simulink model "gm_case2mod_new"  (R2018b)
settings: Solver=FixedStepDiscrete  StartTime=0.0  StopTime=100000  FixedStep=1  RelTol=1e-3
(part 1 of 2)
settings Model: Creator=iris  LastModifiedBy=gvillanova
settings DataIOCC: LimitDataPoints=on  SaveFormat=Array  SignalLoggingSaveFormat=ModelDataLogs  SaveOutput=off  SignalLogging=off  SaveTime=off
settings OptimizationCC: BlockReduction=off  ConditionallyExecuteInputs=off  DefaultParameterBehavior=Inlined  ExpressionDepthLimit=2147483647  LifeSpan=inf
settings DebuggingCC: AlgebraicLoopMsg=error  UnderspecifiedInitializationDetection=Classic  MergeDetectMultiDrivingBlocksExec=none  SolverPrmCheckMsg=warning  InheritedTsInSrcMsg=none  SingleTaskRateTransMsg=error  FcnCallInpInsideContextMsg=warning  StateNameClashWarn=warning  SFUnexpectedBacktrackingDiag=warning  SFNoUnconditionalDefaultTransitionDiag=warning  SFExecutionAtInitializationDiag=none
settings HardwareCC: ProdBitPerPointer=32  ProdBitPerSizeT=32  ProdBitPerPtrDiffT=32  ProdLargestAtomicFloat=None  ProdIntDivRoundTo=Undefined  ProdEndianess=Unspecified  ProdWordSize=32  ProdHWDeviceType=ASIC/FPGA->ASIC/FPGA  ProdEqTarget=off
settings ModelReferenceCC: PropagateSignalLabelsOutOfModel=off
settings SFSimCC: SimUseLocalCustomCode=off
settings RTWCC: RTWUseLocalCustomCode=off
settings CodeAppCC: StateflowObjectComments=on
settings GRTTargetCC: TargetLangStandard=C89/C90 (ANSI)  GeneratePreprocessorConditionals=Disable all  CombineOutputUpdateFcns=off  GRTInterface=on
settings ConfigComp: CovMetricSettings=dw  CovHtmlReporting=on  CovSaveCumulativeToWorkspaceVar=on  CovSaveSingleToWorkspaceVar=on  CovExternalEMLEnable=off

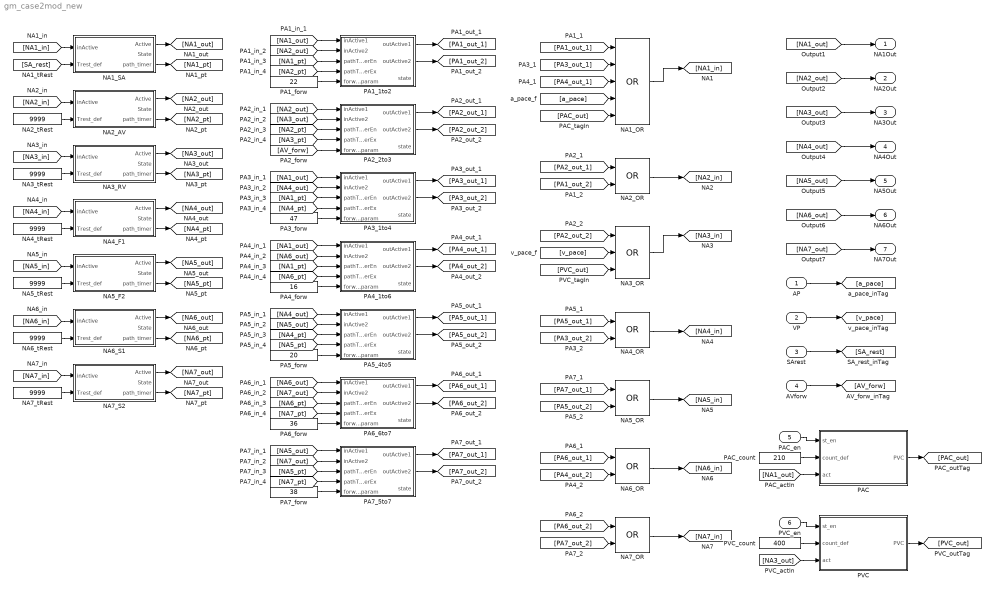
== system gm_case2mod_new ==
  AP : Inport  OutDataTypeStr=boolean  PortDimensions=1  SampleTime=1
  VP : Inport  Port=2  OutDataTypeStr=boolean  PortDimensions=1  SampleTime=1
  SArest : Inport  Port=3  OutDataTypeStr=uint16  PortDimensions=1  SampleTime=1
  AVforw : Inport  Port=4  OutDataTypeStr=uint16  PortDimensions=1  SampleTime=1
  PAC_en : Inport  Port=5  OutDataTypeStr=boolean  PortDimensions=1  SampleTime=1
  PVC_en : Inport  Port=6  OutDataTypeStr=boolean  PortDimensions=1  SampleTime=1
  NA1_OR : Logic  Operator=OR  Inputs=5  AllPortsSameDT=off  OutDataTypeStr=boolean
  NA1_SA : Subsystem  mask{TERP_s_m=double(200), TERP_defs_m=double(200), TRRP_s_m=double(100), TRRP_def_m=double(100), Trest_s_m=double(300), Terp_min_m=double(200), Terp_max_m=double(200)}
      mask prompts: TERP_s_m "Terp Start"; TERP_defs_m "Terp Default Start"; TRRP_s_m "Trrp Start"; TRRP_def_m "Trrp Default"; Trest_s_m "Trest Start"; Terp_min_m "Terp Min"; Terp_max_m "Terp Max"
  NA2_AV : Subsystem  mask{TERP_s_m=double(200), TERP_defs_m=double(200), TRRP_s_m=double(100), TRRP_def_m=double(100), Trest_s_m=double(9999), Terp_min_m=double(200), Terp_max_m=double(200)}
      mask prompts: TERP_s_m "Terp Start"; TERP_defs_m "Terp Default Start"; TRRP_s_m "Trrp Start"; TRRP_def_m "Trrp Default"; Trest_s_m "Trest Start"; Terp_min_m "Terp Min"; Terp_max_m "Terp Max"
  NA2_OR : Logic  Operator=OR  AllPortsSameDT=off  OutDataTypeStr=boolean
  NA2_tRest : Constant  Value=9999  OutDataTypeStr=uint16
  NA3_OR : Logic  Operator=OR  Inputs=3  AllPortsSameDT=off  OutDataTypeStr=boolean
  NA3_RV : Subsystem  mask{TERP_s_m=double(250), TERP_defs_m=double(250), TRRP_s_m=double(100), TRRP_def_m=double(100), Trest_s_m=double(9999), Terp_min_m=double(250), Terp_max_m=double(250)}
      mask prompts: TERP_s_m "Terp Start"; TERP_defs_m "Terp Default Start"; TRRP_s_m "Trrp Start"; TRRP_def_m "Trrp Default"; Trest_s_m "Trest Start"; Terp_min_m "Terp Min"; Terp_max_m "Terp Max"
  NA3_tRest : Constant  Value=9999  OutDataTypeStr=uint16
  NA4_F1 : Subsystem  mask{TERP_s_m=double(250), TERP_defs_m=double(250), TRRP_s_m=double(100), TRRP_def_m=double(100), Trest_s_m=double(9999), Terp_min_m=double(250), Terp_max_m=double(250)}
      mask prompts: TERP_s_m "Terp Start"; TERP_defs_m "Terp Default Start"; TRRP_s_m "Trrp Start"; TRRP_def_m "Trrp Default"; Trest_s_m "Trest Start"; Terp_min_m "Terp Min"; Terp_max_m "Terp Max"
  NA4_OR : Logic  Operator=OR  AllPortsSameDT=off  OutDataTypeStr=boolean
  NA4_tRest : Constant  Value=9999  OutDataTypeStr=uint16
  NA5_F2 : Subsystem  mask{TERP_s_m=double(250), TERP_defs_m=double(250), TRRP_s_m=double(100), TRRP_def_m=double(100), Trest_s_m=double(9999), Terp_min_m=double(250), Terp_max_m=double(250)}
      mask prompts: TERP_s_m "Terp Start"; TERP_defs_m "Terp Default Start"; TRRP_s_m "Trrp Start"; TRRP_def_m "Trrp Default"; Trest_s_m "Trest Start"; Terp_min_m "Terp Min"; Terp_max_m "Terp Max"
  NA5_OR : Logic  Operator=OR  AllPortsSameDT=off  OutDataTypeStr=boolean
  NA5_tRest : Constant  Value=9999  OutDataTypeStr=uint16
  NA6_OR : Logic  Operator=OR  AllPortsSameDT=off  OutDataTypeStr=boolean
  NA6_S1 : Subsystem  mask{TERP_s_m=double(150), TERP_defs_m=double(150), TRRP_s_m=double(100), TRRP_def_m=double(100), Trest_s_m=double(9999), Terp_min_m=double(150), Terp_max_m=double(150)}
      mask prompts: TERP_s_m "Terp Start"; TERP_defs_m "Terp Default Start"; TRRP_s_m "Trrp Start"; TRRP_def_m "Trrp Default"; Trest_s_m "Trest Start"; Terp_min_m "Terp Min"; Terp_max_m "Terp Max"
  NA6_tRest : Constant  Value=9999  OutDataTypeStr=uint16
  NA7_OR : Logic  Operator=OR  AllPortsSameDT=off  OutDataTypeStr=boolean
  NA7_S2 : Subsystem  mask{TERP_s_m=double(150), TERP_defs_m=double(150), TRRP_s_m=double(100), TRRP_def_m=double(100), Trest_s_m=double(9999), Terp_min_m=double(150), Terp_max_m=double(150)}
      mask prompts: TERP_s_m "Terp Start"; TERP_defs_m "Terp Default Start"; TRRP_s_m "Trrp Start"; TRRP_def_m "Trrp Default"; Trest_s_m "Trest Start"; Terp_min_m "Terp Min"; Terp_max_m "Terp Max"
  NA7_tRest : Constant  Value=9999  OutDataTypeStr=uint16
  PA1_1to2 : Subsystem  mask{min_path_par_m=double(10), bck_param_m=double(132)}
      mask prompts: min_path_par_m "Min Path Param"; bck_param_m "Back Param"
  PA1_forw : Constant  Value=22  OutDataTypeStr=uint16
  PA2_2to3 : Subsystem  mask{min_path_par_m=double(90), bck_param_m=double(144)}
      mask prompts: min_path_par_m "Min Path Param"; bck_param_m "Back Param"
  PA3_1to4 : Subsystem  mask{min_path_par_m=double(10), bck_param_m=double(32767)}
      mask prompts: min_path_par_m "Min Path Param"; bck_param_m "Back Param"
  PA3_forw : Constant  Value=47  OutDataTypeStr=uint16
  PA4_1to6 : Subsystem  mask{min_path_par_m=double(80), bck_param_m=double(16)}
      mask prompts: min_path_par_m "Min Path Param"; bck_param_m "Back Param"
  PA4_forw : Constant  Value=16  OutDataTypeStr=uint16
  PA5_4to5 : Subsystem  mask{min_path_par_m=double(50), bck_param_m=double(20)}
      mask prompts: min_path_par_m "Min Path Param"; bck_param_m "Back Param"
  PA5_forw : Constant  Value=20  OutDataTypeStr=uint16
  PA6_6to7 : Subsystem  mask{min_path_par_m=double(100), bck_param_m=double(36)}
      mask prompts: min_path_par_m "Min Path Param"; bck_param_m "Back Param"
  PA6_forw : Constant  Value=36  OutDataTypeStr=uint16
  PA7_5to7 : Subsystem  mask{min_path_par_m=double(50), bck_param_m=double(38)}
      mask prompts: min_path_par_m "Min Path Param"; bck_param_m "Back Param"
  PA7_forw : Constant  Value=38  OutDataTypeStr=uint16
  PAC : Subsystem
  PAC_count : Constant  Value=210  OutDataTypeStr=uint16
  PVC : Subsystem
  PVC_count : Constant  Value=400  OutDataTypeStr=uint16
  NA1Out : Outport
  NA2Out : Outport  Port=2
  NA3Out : Outport  Port=3
  NA4Out : Outport  Port=4
  NA5Out : Outport  Port=5
  NA6Out : Outport  Port=6
  NA7Out : Outport  Port=7
  wires:
  AP/1 -> [a_pace]
  VP/1 -> [v_pace]
  SArest/1 -> [SA_rest]
  AVforw/1 -> [AV_forw]
  PAC_en/1 -> PAC/1(st_en)
  PVC_en/1 -> PVC/1(st_en)
  NA1_OR/1 -> [NA1_in]
  NA1_SA/1(Active) -> [NA1_out]
  NA1_SA/3(path_timer) -> [NA1_pt]
  [NA1_in] -> NA1_SA/1(inActive)
  [SA_rest] -> NA1_SA/2(Trest_def)
  NA2_AV/1(Active) -> [NA2_out]
  NA2_AV/3(path_timer) -> [NA2_pt]
  NA2_OR/1 -> [NA2_in]
  [NA2_in] -> NA2_AV/1(inActive)
  NA2_tRest/1 -> NA2_AV/2(Trest_def)
  NA3_OR/1 -> [NA3_in]
  NA3_RV/1(Active) -> [NA3_out]
  NA3_RV/3(path_timer) -> [NA3_pt]
  [NA3_in] -> NA3_RV/1(inActive)
  NA3_tRest/1 -> NA3_RV/2(Trest_def)
  NA4_F1/1(Active) -> [NA4_out]
  NA4_F1/3(path_timer) -> [NA4_pt]
  NA4_OR/1 -> [NA4_in]
  [NA4_in] -> NA4_F1/1(inActive)
  NA4_tRest/1 -> NA4_F1/2(Trest_def)
  NA5_F2/1(Active) -> [NA5_out]
  NA5_F2/3(path_timer) -> [NA5_pt]
  NA5_OR/1 -> [NA5_in]
  [NA5_in] -> NA5_F2/1(inActive)
  NA5_tRest/1 -> NA5_F2/2(Trest_def)
  NA6_OR/1 -> [NA6_in]
  NA6_S1/1(Active) -> [NA6_out]
  NA6_S1/3(path_timer) -> [NA6_pt]
  [NA6_in] -> NA6_S1/1(inActive)
  NA6_tRest/1 -> NA6_S1/2(Trest_def)
  NA7_OR/1 -> [NA7_in]
  NA7_S2/1(Active) -> [NA7_out]
  NA7_S2/3(path_timer) -> [NA7_pt]
  [NA7_in] -> NA7_S2/1(inActive)
  NA7_tRest/1 -> NA7_S2/2(Trest_def)
  [NA1_out] -> NA1Out/1
  [NA2_out] -> NA2Out/1
  [NA3_out] -> NA3Out/1
  [NA4_out] -> NA4Out/1
  [NA5_out] -> NA5Out/1
  [NA6_out] -> NA6Out/1
  [NA7_out] -> NA7Out/1
  [PA1_out_1] -> NA1_OR/1
  PA1_1to2/1(outActive1) -> [PA1_out_1]
  PA1_1to2/2(outActive2) -> [PA1_out_2]
  [PA1_out_2] -> NA2_OR/2
  PA1_forw/1 -> PA1_1to2/5(forw_param)
  [NA1_out] -> PA1_1to2/1(inActive1)
  [NA2_out] -> PA1_1to2/2(inActive2)
  [NA1_pt] -> PA1_1to2/3(pathTimerEn)
  [NA2_pt] -> PA1_1to2/4(pathTimerEx)
  [PA2_out_1] -> NA2_OR/1
  [PA2_out_2] -> NA3_OR/1
  PA2_2to3/1(outActive1) -> [PA2_out_1]
  PA2_2to3/2(outActive2) -> [PA2_out_2]
  [AV_forw] -> PA2_2to3/5(forw_param)
  [NA2_out] -> PA2_2to3/1(inActive1)
  [NA3_out] -> PA2_2to3/2(inActive2)
  [NA2_pt] -> PA2_2to3/3(pathTimerEn)
  [NA3_pt] -> PA2_2to3/4(pathTimerEx)
  [PA3_out_1] -> NA1_OR/2
  PA3_1to4/1(outActive1) -> [PA3_out_1]
  PA3_1to4/2(outActive2) -> [PA3_out_2]
  [PA3_out_2] -> NA4_OR/2
  PA3_forw/1 -> PA3_1to4/5(forw_param)
  [NA1_out] -> PA3_1to4/1(inActive1)
  [NA4_out] -> PA3_1to4/2(inActive2)
  [NA1_pt] -> PA3_1to4/3(pathTimerEn)
  [NA4_pt] -> PA3_1to4/4(pathTimerEx)
  [PA4_out_1] -> NA1_OR/3
  PA4_1to6/1(outActive1) -> [PA4_out_1]
  PA4_1to6/2(outActive2) -> [PA4_out_2]
  [PA4_out_2] -> NA6_OR/2
  PA4_forw/1 -> PA4_1to6/5(forw_param)
  [NA1_out] -> PA4_1to6/1(inActive1)
  [NA6_out] -> PA4_1to6/2(inActive2)
  [NA1_pt] -> PA4_1to6/3(pathTimerEn)
  [NA6_pt] -> PA4_1to6/4(pathTimerEx)
  [PA5_out_1] -> NA4_OR/1
  [PA5_out_2] -> NA5_OR/2
  PA5_4to5/1(outActive1) -> [PA5_out_1]
  PA5_4to5/2(outActive2) -> [PA5_out_2]
  PA5_forw/1 -> PA5_4to5/5(forw_param)
  [NA4_out] -> PA5_4to5/1(inActive1)
  [NA5_out] -> PA5_4to5/2(inActive2)
  [NA4_pt] -> PA5_4to5/3(pathTimerEn)
  [NA5_pt] -> PA5_4to5/4(pathTimerEx)
  [PA6_out_1] -> NA6_OR/1
  [PA6_out_2] -> NA7_OR/1
  PA6_6to7/1(outActive1) -> [PA6_out_1]
  PA6_6to7/2(outActive2) -> [PA6_out_2]
  PA6_forw/1 -> PA6_6to7/5(forw_param)
  [NA6_out] -> PA6_6to7/1(inActive1)
  [NA7_out] -> PA6_6to7/2(inActive2)
  [NA6_pt] -> PA6_6to7/3(pathTimerEn)
  [NA7_pt] -> PA6_6to7/4(pathTimerEx)
  [PA7_out_1] -> NA5_OR/1
  [PA7_out_2] -> NA7_OR/2
  PA7_5to7/1(outActive1) -> [PA7_out_1]
  PA7_5to7/2(outActive2) -> [PA7_out_2]
  PA7_forw/1 -> PA7_5to7/5(forw_param)
  [NA5_out] -> PA7_5to7/1(inActive1)
  [NA7_out] -> PA7_5to7/2(inActive2)
  [NA5_pt] -> PA7_5to7/3(pathTimerEn)
  [NA7_pt] -> PA7_5to7/4(pathTimerEx)
  PAC/1(PVC) -> [PAC_out]
  [NA1_out] -> PAC/3(act)
  PAC_count/1 -> PAC/2(count_def)
  [PAC_out] -> NA1_OR/5
  PVC/1(PVC) -> [PVC_out]
  [NA3_out] -> PVC/3(act)
  PVC_count/1 -> PVC/2(count_def)
  [PVC_out] -> NA3_OR/3
  [a_pace] -> NA1_OR/4
  [v_pace] -> NA3_OR/2

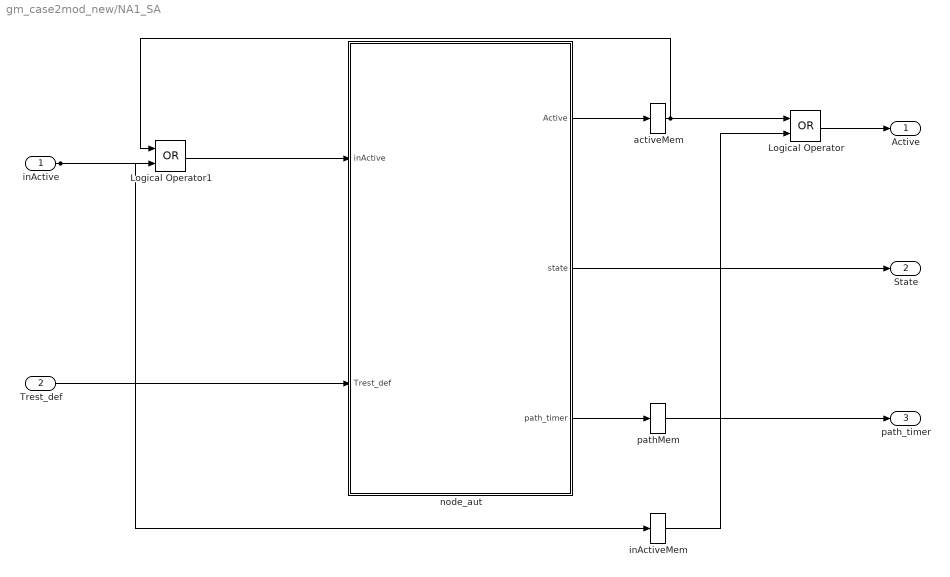
== system gm_case2mod_new/NA1_SA ==
  inActive : Inport  OutDataTypeStr=boolean  SampleTime=1
  Trest_def : Inport  Port=2  OutDataTypeStr=uint16  SampleTime=1
  Logical Operator : Logic  Operator=OR  AllPortsSameDT=off  OutDataTypeStr=boolean
  Logical Operator1 : Logic  Operator=OR  AllPortsSameDT=off  OutDataTypeStr=boolean
  activeMem : Memory  InheritSampleTime=on
  inActiveMem : Memory  InheritSampleTime=on
  node_aut : Subsystem
  pathMem : Memory  InheritSampleTime=on
  Active : Outport
  State : Outport  Port=2
  path_timer : Outport  Port=3
  wires:
  inActive/1 -> Logical Operator1/2, inActiveMem/1
  Trest_def/1 -> node_aut/2(Trest_def)
  Logical Operator/1 -> Active/1
  Logical Operator1/1 -> node_aut/1(inActive)
  activeMem/1 -> Logical Operator1/1, Logical Operator/1
  inActiveMem/1 -> Logical Operator/2
  node_aut/1(Active) -> activeMem/1
  node_aut/2(state) -> State/1
  node_aut/3(path_timer) -> pathMem/1
  pathMem/1 -> path_timer/1

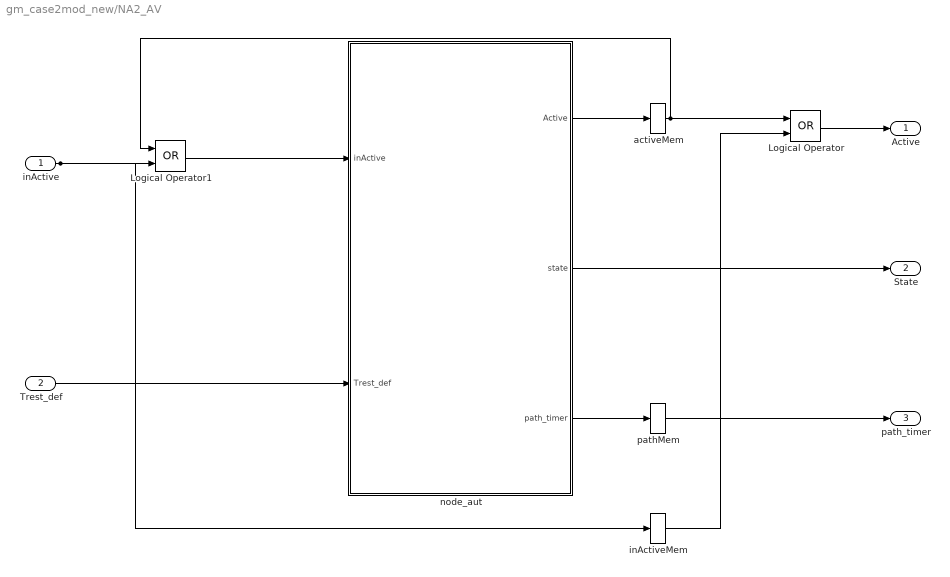
== system gm_case2mod_new/NA2_AV ==
  inActive : Inport  OutDataTypeStr=boolean  SampleTime=1
  Trest_def : Inport  Port=2  OutDataTypeStr=uint16
  Logical Operator : Logic  Operator=OR  AllPortsSameDT=off  OutDataTypeStr=boolean
  Logical Operator1 : Logic  Operator=OR  AllPortsSameDT=off  OutDataTypeStr=boolean
  activeMem : Memory  InheritSampleTime=on
  inActiveMem : Memory  InheritSampleTime=on
  node_aut : Subsystem
  pathMem : Memory  InheritSampleTime=on
  Active : Outport
  State : Outport  Port=2
  path_timer : Outport  Port=3
  wires:
  inActive/1 -> Logical Operator1/2, inActiveMem/1
  Trest_def/1 -> node_aut/2(Trest_def)
  Logical Operator/1 -> Active/1
  Logical Operator1/1 -> node_aut/1(inActive)
  activeMem/1 -> Logical Operator1/1, Logical Operator/1
  inActiveMem/1 -> Logical Operator/2
  node_aut/1(Active) -> activeMem/1
  node_aut/2(state) -> State/1
  node_aut/3(path_timer) -> pathMem/1
  pathMem/1 -> path_timer/1

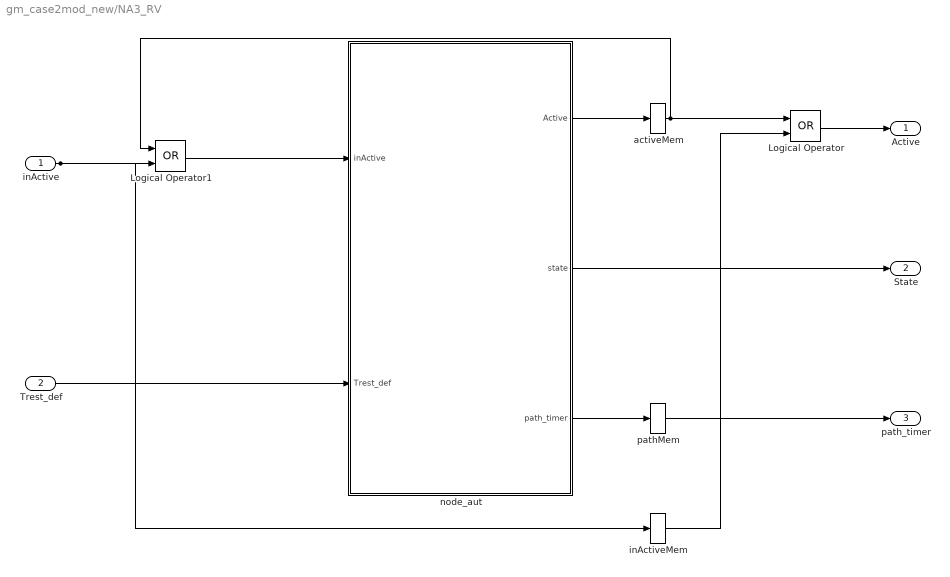
== system gm_case2mod_new/NA3_RV ==
  inActive : Inport  OutDataTypeStr=boolean  SampleTime=1
  Trest_def : Inport  Port=2  OutDataTypeStr=uint16
  Logical Operator : Logic  Operator=OR  AllPortsSameDT=off  OutDataTypeStr=boolean
  Logical Operator1 : Logic  Operator=OR  AllPortsSameDT=off  OutDataTypeStr=boolean
  activeMem : Memory  InheritSampleTime=on
  inActiveMem : Memory  InheritSampleTime=on
  node_aut : Subsystem
  pathMem : Memory  InheritSampleTime=on
  Active : Outport
  State : Outport  Port=2
  path_timer : Outport  Port=3
  wires:
  inActive/1 -> Logical Operator1/2, inActiveMem/1
  Trest_def/1 -> node_aut/2(Trest_def)
  Logical Operator/1 -> Active/1
  Logical Operator1/1 -> node_aut/1(inActive)
  activeMem/1 -> Logical Operator1/1, Logical Operator/1
  inActiveMem/1 -> Logical Operator/2
  node_aut/1(Active) -> activeMem/1
  node_aut/2(state) -> State/1
  node_aut/3(path_timer) -> pathMem/1
  pathMem/1 -> path_timer/1

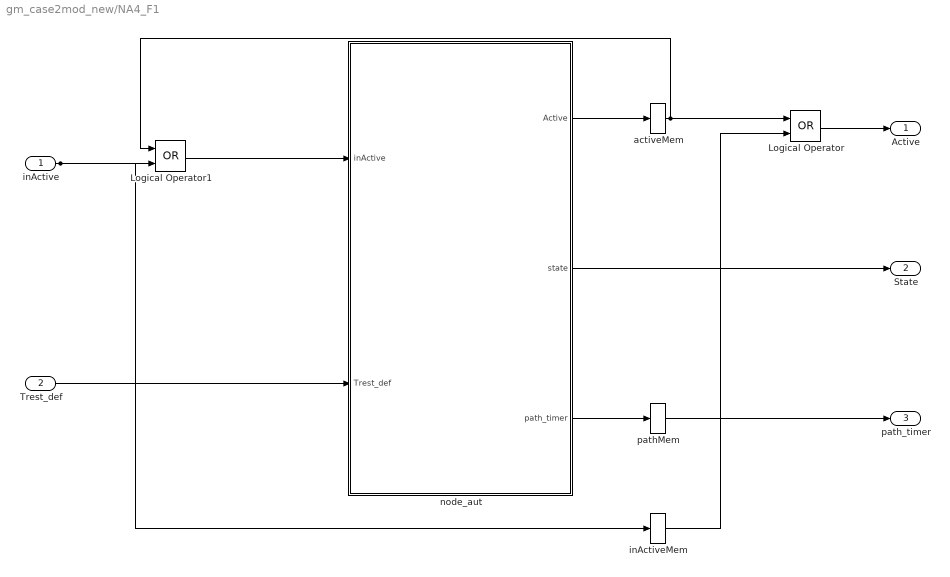
== system gm_case2mod_new/NA4_F1 ==
  inActive : Inport  OutDataTypeStr=boolean  SampleTime=1
  Trest_def : Inport  Port=2  OutDataTypeStr=uint16
  Logical Operator : Logic  Operator=OR  AllPortsSameDT=off  OutDataTypeStr=boolean
  Logical Operator1 : Logic  Operator=OR  AllPortsSameDT=off  OutDataTypeStr=boolean
  activeMem : Memory  InheritSampleTime=on
  inActiveMem : Memory  InheritSampleTime=on
  node_aut : Subsystem
  pathMem : Memory  InheritSampleTime=on
  Active : Outport
  State : Outport  Port=2
  path_timer : Outport  Port=3
  wires:
  inActive/1 -> Logical Operator1/2, inActiveMem/1
  Trest_def/1 -> node_aut/2(Trest_def)
  Logical Operator/1 -> Active/1
  Logical Operator1/1 -> node_aut/1(inActive)
  activeMem/1 -> Logical Operator1/1, Logical Operator/1
  inActiveMem/1 -> Logical Operator/2
  node_aut/1(Active) -> activeMem/1
  node_aut/2(state) -> State/1
  node_aut/3(path_timer) -> pathMem/1
  pathMem/1 -> path_timer/1

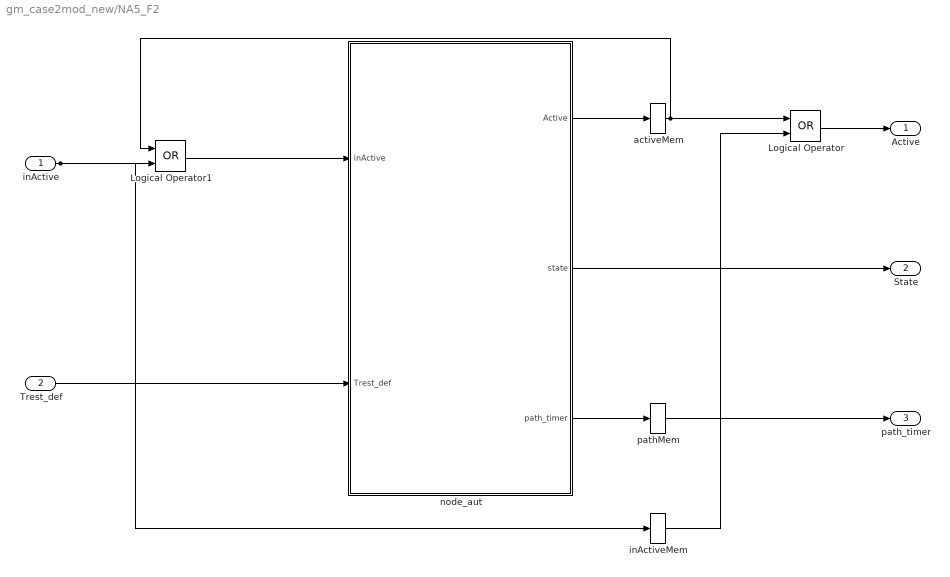
== system gm_case2mod_new/NA5_F2 ==
  inActive : Inport  OutDataTypeStr=boolean  SampleTime=1
  Trest_def : Inport  Port=2  OutDataTypeStr=uint16
  Logical Operator : Logic  Operator=OR  AllPortsSameDT=off  OutDataTypeStr=boolean
  Logical Operator1 : Logic  Operator=OR  AllPortsSameDT=off  OutDataTypeStr=boolean
  activeMem : Memory  InheritSampleTime=on
  inActiveMem : Memory  InheritSampleTime=on
  node_aut : Subsystem
  pathMem : Memory  InheritSampleTime=on
  Active : Outport
  State : Outport  Port=2
  path_timer : Outport  Port=3
  wires:
  inActive/1 -> Logical Operator1/2, inActiveMem/1
  Trest_def/1 -> node_aut/2(Trest_def)
  Logical Operator/1 -> Active/1
  Logical Operator1/1 -> node_aut/1(inActive)
  activeMem/1 -> Logical Operator1/1, Logical Operator/1
  inActiveMem/1 -> Logical Operator/2
  node_aut/1(Active) -> activeMem/1
  node_aut/2(state) -> State/1
  node_aut/3(path_timer) -> pathMem/1
  pathMem/1 -> path_timer/1

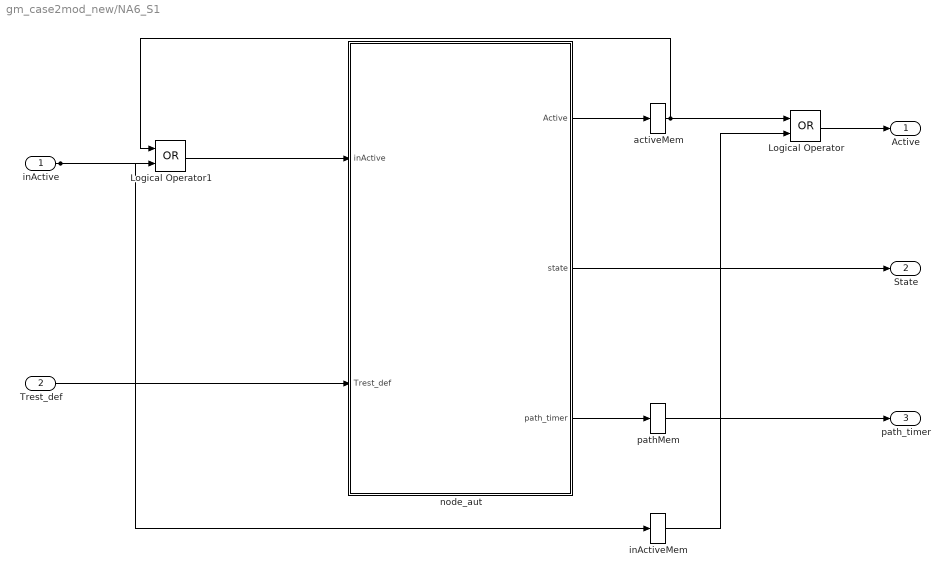
== system gm_case2mod_new/NA6_S1 ==
  inActive : Inport  OutDataTypeStr=boolean  SampleTime=1
  Trest_def : Inport  Port=2  OutDataTypeStr=uint16
  Logical Operator : Logic  Operator=OR  AllPortsSameDT=off  OutDataTypeStr=boolean
  Logical Operator1 : Logic  Operator=OR  AllPortsSameDT=off  OutDataTypeStr=boolean
  activeMem : Memory  InheritSampleTime=on
  inActiveMem : Memory  InheritSampleTime=on
  node_aut : Subsystem
  pathMem : Memory  InheritSampleTime=on
  Active : Outport
  State : Outport  Port=2
  path_timer : Outport  Port=3
  wires:
  inActive/1 -> Logical Operator1/2, inActiveMem/1
  Trest_def/1 -> node_aut/2(Trest_def)
  Logical Operator/1 -> Active/1
  Logical Operator1/1 -> node_aut/1(inActive)
  activeMem/1 -> Logical Operator1/1, Logical Operator/1
  inActiveMem/1 -> Logical Operator/2
  node_aut/1(Active) -> activeMem/1
  node_aut/2(state) -> State/1
  node_aut/3(path_timer) -> pathMem/1
  pathMem/1 -> path_timer/1

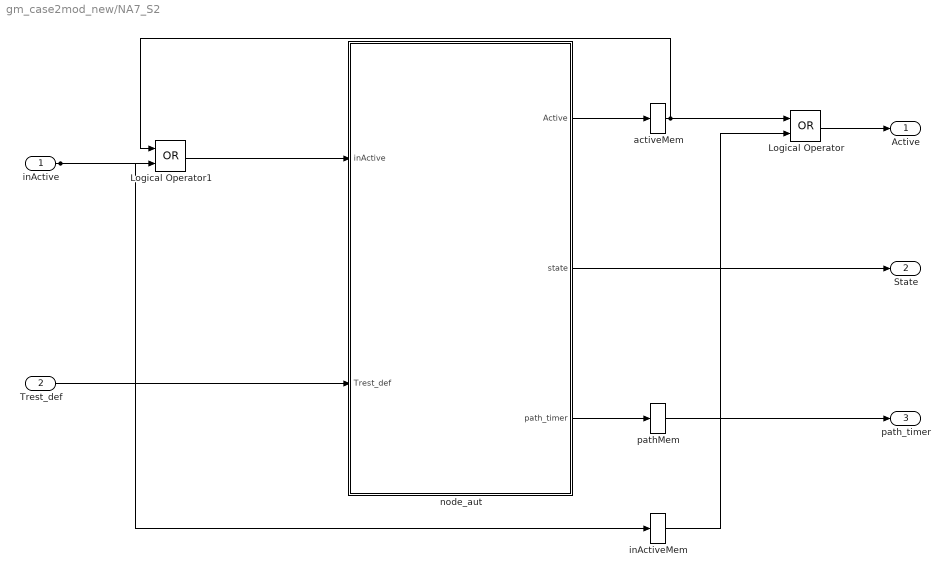
== system gm_case2mod_new/NA7_S2 ==
  inActive : Inport  OutDataTypeStr=boolean  SampleTime=1
  Trest_def : Inport  Port=2  OutDataTypeStr=uint16
  Logical Operator : Logic  Operator=OR  AllPortsSameDT=off  OutDataTypeStr=boolean
  Logical Operator1 : Logic  Operator=OR  AllPortsSameDT=off  OutDataTypeStr=boolean
  activeMem : Memory  InheritSampleTime=on
  inActiveMem : Memory  InheritSampleTime=on
  node_aut : Subsystem
  pathMem : Memory  InheritSampleTime=on
  Active : Outport
  State : Outport  Port=2
  path_timer : Outport  Port=3
  wires:
  inActive/1 -> Logical Operator1/2, inActiveMem/1
  Trest_def/1 -> node_aut/2(Trest_def)
  Logical Operator/1 -> Active/1
  Logical Operator1/1 -> node_aut/1(inActive)
  activeMem/1 -> Logical Operator1/1, Logical Operator/1
  inActiveMem/1 -> Logical Operator/2
  node_aut/1(Active) -> activeMem/1
  node_aut/2(state) -> State/1
  node_aut/3(path_timer) -> pathMem/1
  pathMem/1 -> path_timer/1

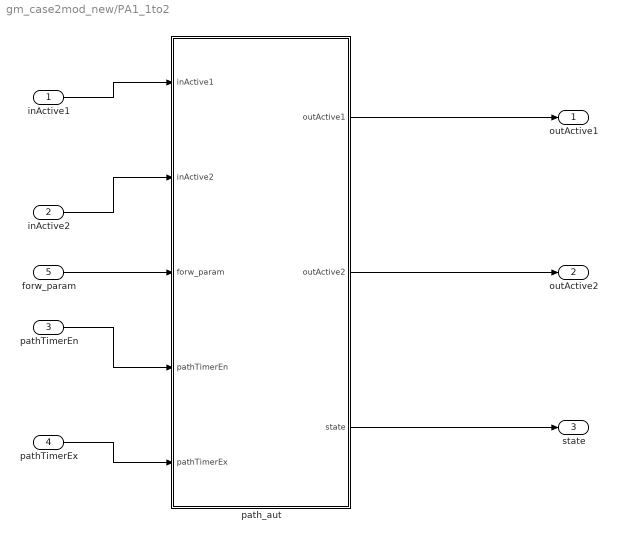
== system gm_case2mod_new/PA1_1to2 ==
  inActive1 : Inport  OutDataTypeStr=boolean  SampleTime=1
  inActive2 : Inport  Port=2  OutDataTypeStr=boolean  SampleTime=1
  pathTimerEn : Inport  Port=3  OutDataTypeStr=uint16  SampleTime=1
  pathTimerEx : Inport  Port=4  OutDataTypeStr=uint16  SampleTime=1
  forw_param : Inport  Port=5  OutDataTypeStr=uint16
  path_aut : Subsystem
  outActive1 : Outport
  outActive2 : Outport  Port=2
  state : Outport  Port=3
  wires:
  inActive1/1 -> path_aut/1(inActive1)
  inActive2/1 -> path_aut/2(inActive2)
  pathTimerEn/1 -> path_aut/4(pathTimerEn)
  pathTimerEx/1 -> path_aut/5(pathTimerEx)
  forw_param/1 -> path_aut/3(forw_param)
  path_aut/1(outActive1) -> outActive1/1
  path_aut/2(outActive2) -> outActive2/1
  path_aut/3(state) -> state/1

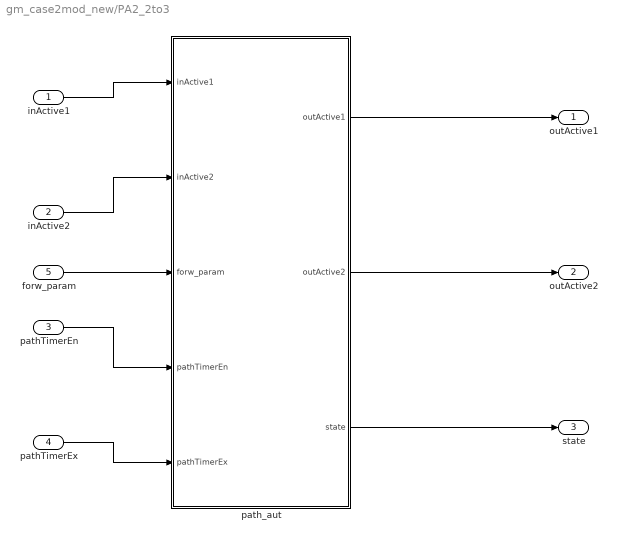
== system gm_case2mod_new/PA2_2to3 ==
  inActive1 : Inport  OutDataTypeStr=boolean  SampleTime=1
  inActive2 : Inport  Port=2  OutDataTypeStr=boolean  SampleTime=1
  pathTimerEn : Inport  Port=3  OutDataTypeStr=uint16  SampleTime=1
  pathTimerEx : Inport  Port=4  OutDataTypeStr=uint16  SampleTime=1
  forw_param : Inport  Port=5  OutDataTypeStr=uint16  SampleTime=1
  path_aut : Subsystem
  outActive1 : Outport
  outActive2 : Outport  Port=2
  state : Outport  Port=3
  wires:
  inActive1/1 -> path_aut/1(inActive1)
  inActive2/1 -> path_aut/2(inActive2)
  pathTimerEn/1 -> path_aut/4(pathTimerEn)
  pathTimerEx/1 -> path_aut/5(pathTimerEx)
  forw_param/1 -> path_aut/3(forw_param)
  path_aut/1(outActive1) -> outActive1/1
  path_aut/2(outActive2) -> outActive2/1
  path_aut/3(state) -> state/1

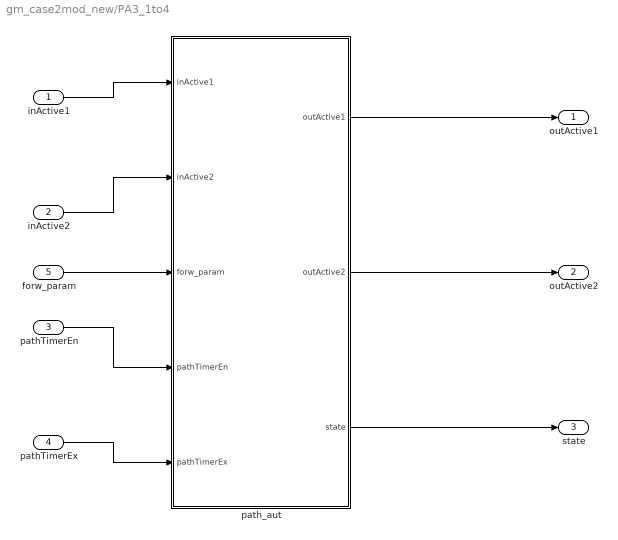
== system gm_case2mod_new/PA3_1to4 ==
  inActive1 : Inport  OutDataTypeStr=boolean  SampleTime=1
  inActive2 : Inport  Port=2  OutDataTypeStr=boolean  SampleTime=1
  pathTimerEn : Inport  Port=3  OutDataTypeStr=uint16  SampleTime=1
  pathTimerEx : Inport  Port=4  OutDataTypeStr=uint16  SampleTime=1
  forw_param : Inport  Port=5  OutDataTypeStr=uint16
  path_aut : Subsystem
  outActive1 : Outport
  outActive2 : Outport  Port=2
  state : Outport  Port=3
  wires:
  inActive1/1 -> path_aut/1(inActive1)
  inActive2/1 -> path_aut/2(inActive2)
  pathTimerEn/1 -> path_aut/4(pathTimerEn)
  pathTimerEx/1 -> path_aut/5(pathTimerEx)
  forw_param/1 -> path_aut/3(forw_param)
  path_aut/1(outActive1) -> outActive1/1
  path_aut/2(outActive2) -> outActive2/1
  path_aut/3(state) -> state/1

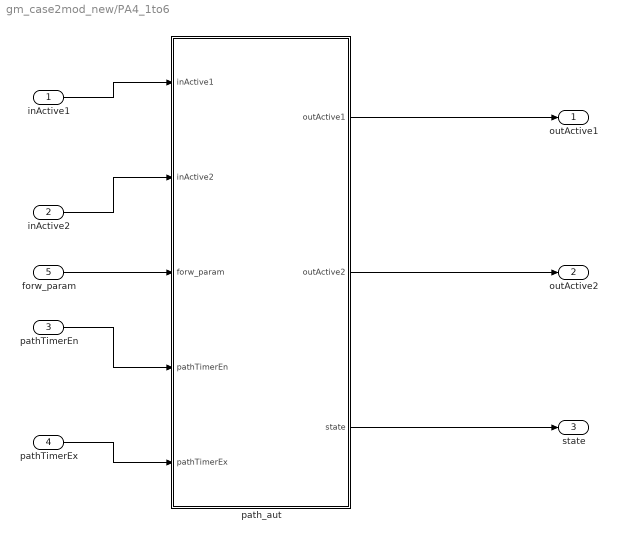
== system gm_case2mod_new/PA4_1to6 ==
  inActive1 : Inport  OutDataTypeStr=boolean  SampleTime=1
  inActive2 : Inport  Port=2  OutDataTypeStr=boolean  SampleTime=1
  pathTimerEn : Inport  Port=3  OutDataTypeStr=uint16  SampleTime=1
  pathTimerEx : Inport  Port=4  OutDataTypeStr=uint16  SampleTime=1
  forw_param : Inport  Port=5  OutDataTypeStr=uint16
  path_aut : Subsystem
  outActive1 : Outport
  outActive2 : Outport  Port=2
  state : Outport  Port=3
  wires:
  inActive1/1 -> path_aut/1(inActive1)
  inActive2/1 -> path_aut/2(inActive2)
  pathTimerEn/1 -> path_aut/4(pathTimerEn)
  pathTimerEx/1 -> path_aut/5(pathTimerEx)
  forw_param/1 -> path_aut/3(forw_param)
  path_aut/1(outActive1) -> outActive1/1
  path_aut/2(outActive2) -> outActive2/1
  path_aut/3(state) -> state/1

== system gm_case2mod_new/PA5_4to5 ==
  inActive1 : Inport  OutDataTypeStr=boolean  SampleTime=1
  inActive2 : Inport  Port=2  OutDataTypeStr=boolean  SampleTime=1
  pathTimerEn : Inport  Port=3  OutDataTypeStr=uint16  SampleTime=1
  pathTimerEx : Inport  Port=4  OutDataTypeStr=uint16  SampleTime=1
  forw_param : Inport  Port=5  OutDataTypeStr=uint16
  path_aut : Subsystem
  outActive1 : Outport
  outActive2 : Outport  Port=2
  state : Outport  Port=3
  wires:
  inActive1/1 -> path_aut/1(inActive1)
  inActive2/1 -> path_aut/2(inActive2)
  pathTimerEn/1 -> path_aut/4(pathTimerEn)
  pathTimerEx/1 -> path_aut/5(pathTimerEx)
  forw_param/1 -> path_aut/3(forw_param)
  path_aut/1(outActive1) -> outActive1/1
  path_aut/2(outActive2) -> outActive2/1
  path_aut/3(state) -> state/1

== system gm_case2mod_new/PA6_6to7 ==
  inActive1 : Inport  OutDataTypeStr=boolean  SampleTime=1
  inActive2 : Inport  Port=2  OutDataTypeStr=boolean  SampleTime=1
  pathTimerEn : Inport  Port=3  OutDataTypeStr=uint16  SampleTime=1
  pathTimerEx : Inport  Port=4  OutDataTypeStr=uint16  SampleTime=1
  forw_param : Inport  Port=5  OutDataTypeStr=uint16
  path_aut : Subsystem
  outActive1 : Outport
  outActive2 : Outport  Port=2
  state : Outport  Port=3
  wires:
  inActive1/1 -> path_aut/1(inActive1)
  inActive2/1 -> path_aut/2(inActive2)
  pathTimerEn/1 -> path_aut/4(pathTimerEn)
  pathTimerEx/1 -> path_aut/5(pathTimerEx)
  forw_param/1 -> path_aut/3(forw_param)
  path_aut/1(outActive1) -> outActive1/1
  path_aut/2(outActive2) -> outActive2/1
  path_aut/3(state) -> state/1

== system gm_case2mod_new/PA7_5to7 ==
  inActive1 : Inport  OutDataTypeStr=boolean  SampleTime=1
  inActive2 : Inport  Port=2  OutDataTypeStr=boolean  SampleTime=1
  pathTimerEn : Inport  Port=3  OutDataTypeStr=uint16  SampleTime=1
  pathTimerEx : Inport  Port=4  OutDataTypeStr=uint16  SampleTime=1
  forw_param : Inport  Port=5  OutDataTypeStr=uint16
  path_aut : Subsystem
  outActive1 : Outport
  outActive2 : Outport  Port=2
  state : Outport  Port=3
  wires:
  inActive1/1 -> path_aut/1(inActive1)
  inActive2/1 -> path_aut/2(inActive2)
  pathTimerEn/1 -> path_aut/4(pathTimerEn)
  pathTimerEx/1 -> path_aut/5(pathTimerEx)
  forw_param/1 -> path_aut/3(forw_param)
  path_aut/1(outActive1) -> outActive1/1
  path_aut/2(outActive2) -> outActive2/1
  path_aut/3(state) -> state/1

== system gm_case2mod_new/PAC ==
  st_en : Inport  OutDataTypeStr=boolean  SampleTime=1
  count_def : Inport  Port=2  OutDataTypeStr=uint16
  act : Inport  Port=3  OutDataTypeStr=boolean  SampleTime=1
  SimpleModeling_c8_PVC : Stateflow chart  TreatAsAtomicUnit=on
  PVC : Outport
  wires:
  st_en/1 -> SimpleModeling_c8_PVC/1(st_en)
  count_def/1 -> SimpleModeling_c8_PVC/2(count_def)
  act/1 -> SimpleModeling_c8_PVC/3(act)
  SimpleModeling_c8_PVC/1(PVC) -> PVC/1

== system gm_case2mod_new/PVC ==
  st_en : Inport  OutDataTypeStr=boolean  SampleTime=1
  count_def : Inport  Port=2  OutDataTypeStr=uint16
  act : Inport  Port=3  OutDataTypeStr=boolean  SampleTime=1
  SimpleModeling_c8_PVC : Stateflow chart  TreatAsAtomicUnit=on
  PVC : Outport
  wires:
  SimpleModeling_c8_PVC/1(PVC) -> PVC/1
  act/1 -> SimpleModeling_c8_PVC/3(act)
  count_def/1 -> SimpleModeling_c8_PVC/2(count_def)
  st_en/1 -> SimpleModeling_c8_PVC/1(st_en)

== system gm_case2mod_new/NA1_SA/node_aut ==
  inActive : Inport  OutDataTypeStr=boolean  PortDimensions=1  SampleTime=1
  Trest_def : Inport  Port=2  OutDataTypeStr=uint16  PortDimensions=1  SampleTime=1
  SimpleModeling_c4_srNoRdC9XVw08QQmbgBst2F_node_aut : Stateflow chart  TreatAsAtomicUnit=on
  Active : Outport
  state : Outport  Port=2
  path_timer : Outport  Port=3
  wires:
  inActive/1 -> SimpleModeling_c4_srNoRdC9XVw08QQmbgBst2F_node_aut/1(inActive)
  Trest_def/1 -> SimpleModeling_c4_srNoRdC9XVw08QQmbgBst2F_node_aut/2(Trest_def)
  SimpleModeling_c4_srNoRdC9XVw08QQmbgBst2F_node_aut/1(Active) -> Active/1
  SimpleModeling_c4_srNoRdC9XVw08QQmbgBst2F_node_aut/2(state) -> state/1
  SimpleModeling_c4_srNoRdC9XVw08QQmbgBst2F_node_aut/3(path_timer) -> path_timer/1

== system gm_case2mod_new/NA2_AV/node_aut ==
  inActive : Inport  OutDataTypeStr=boolean  PortDimensions=1  SampleTime=1
  Trest_def : Inport  Port=2  OutDataTypeStr=uint16  PortDimensions=1
  SimpleModeling_c4_sQ0mRpZY21gn33BKqBQ1TvG_node_aut : Stateflow chart  TreatAsAtomicUnit=on
  Active : Outport
  state : Outport  Port=2
  path_timer : Outport  Port=3
  wires:
  inActive/1 -> SimpleModeling_c4_sQ0mRpZY21gn33BKqBQ1TvG_node_aut/1(inActive)
  Trest_def/1 -> SimpleModeling_c4_sQ0mRpZY21gn33BKqBQ1TvG_node_aut/2(Trest_def)
  SimpleModeling_c4_sQ0mRpZY21gn33BKqBQ1TvG_node_aut/1(Active) -> Active/1
  SimpleModeling_c4_sQ0mRpZY21gn33BKqBQ1TvG_node_aut/2(state) -> state/1
  SimpleModeling_c4_sQ0mRpZY21gn33BKqBQ1TvG_node_aut/3(path_timer) -> path_timer/1

== system gm_case2mod_new/NA3_RV/node_aut ==
  inActive : Inport  OutDataTypeStr=boolean  PortDimensions=1  SampleTime=1
  Trest_def : Inport  Port=2  OutDataTypeStr=uint16  PortDimensions=1
  SimpleModeling_c4_sppf4LupdbMSnBPpv0jGkfF_node_aut : Stateflow chart  TreatAsAtomicUnit=on
  Active : Outport
  state : Outport  Port=2
  path_timer : Outport  Port=3
  wires:
  inActive/1 -> SimpleModeling_c4_sppf4LupdbMSnBPpv0jGkfF_node_aut/1(inActive)
  Trest_def/1 -> SimpleModeling_c4_sppf4LupdbMSnBPpv0jGkfF_node_aut/2(Trest_def)
  SimpleModeling_c4_sppf4LupdbMSnBPpv0jGkfF_node_aut/1(Active) -> Active/1
  SimpleModeling_c4_sppf4LupdbMSnBPpv0jGkfF_node_aut/2(state) -> state/1
  SimpleModeling_c4_sppf4LupdbMSnBPpv0jGkfF_node_aut/3(path_timer) -> path_timer/1

== system gm_case2mod_new/NA4_F1/node_aut ==
  inActive : Inport  OutDataTypeStr=boolean  PortDimensions=1  SampleTime=1
  Trest_def : Inport  Port=2  OutDataTypeStr=uint16  PortDimensions=1
  SimpleModeling_c4_sppf4LupdbMSnBPpv0jGkfF_node_aut : Stateflow chart  TreatAsAtomicUnit=on
  Active : Outport
  state : Outport  Port=2
  path_timer : Outport  Port=3
  wires:
  SimpleModeling_c4_sppf4LupdbMSnBPpv0jGkfF_node_aut/3(path_timer) -> path_timer/1
  SimpleModeling_c4_sppf4LupdbMSnBPpv0jGkfF_node_aut/2(state) -> state/1
  SimpleModeling_c4_sppf4LupdbMSnBPpv0jGkfF_node_aut/1(Active) -> Active/1
  Trest_def/1 -> SimpleModeling_c4_sppf4LupdbMSnBPpv0jGkfF_node_aut/2(Trest_def)
  inActive/1 -> SimpleModeling_c4_sppf4LupdbMSnBPpv0jGkfF_node_aut/1(inActive)

== system gm_case2mod_new/NA5_F2/node_aut ==
  inActive : Inport  OutDataTypeStr=boolean  PortDimensions=1  SampleTime=1
  Trest_def : Inport  Port=2  OutDataTypeStr=uint16  PortDimensions=1
  SimpleModeling_c4_sppf4LupdbMSnBPpv0jGkfF_node_aut : Stateflow chart  TreatAsAtomicUnit=on
  Active : Outport
  state : Outport  Port=2
  path_timer : Outport  Port=3
  wires:
  SimpleModeling_c4_sppf4LupdbMSnBPpv0jGkfF_node_aut/3(path_timer) -> path_timer/1
  SimpleModeling_c4_sppf4LupdbMSnBPpv0jGkfF_node_aut/2(state) -> state/1
  SimpleModeling_c4_sppf4LupdbMSnBPpv0jGkfF_node_aut/1(Active) -> Active/1
  Trest_def/1 -> SimpleModeling_c4_sppf4LupdbMSnBPpv0jGkfF_node_aut/2(Trest_def)
  inActive/1 -> SimpleModeling_c4_sppf4LupdbMSnBPpv0jGkfF_node_aut/1(inActive)

== system gm_case2mod_new/NA6_S1/node_aut ==
  inActive : Inport  OutDataTypeStr=boolean  PortDimensions=1  SampleTime=1
  Trest_def : Inport  Port=2  OutDataTypeStr=uint16  PortDimensions=1
  SimpleModeling_c4_sqCkIiGJ54r4u5oiueanYzC_node_aut : Stateflow chart  TreatAsAtomicUnit=on
  Active : Outport
  state : Outport  Port=2
  path_timer : Outport  Port=3
  wires:
  inActive/1 -> SimpleModeling_c4_sqCkIiGJ54r4u5oiueanYzC_node_aut/1(inActive)
  Trest_def/1 -> SimpleModeling_c4_sqCkIiGJ54r4u5oiueanYzC_node_aut/2(Trest_def)
  SimpleModeling_c4_sqCkIiGJ54r4u5oiueanYzC_node_aut/1(Active) -> Active/1
  SimpleModeling_c4_sqCkIiGJ54r4u5oiueanYzC_node_aut/2(state) -> state/1
  SimpleModeling_c4_sqCkIiGJ54r4u5oiueanYzC_node_aut/3(path_timer) -> path_timer/1

== system gm_case2mod_new/NA7_S2/node_aut ==
  inActive : Inport  OutDataTypeStr=boolean  PortDimensions=1  SampleTime=1
  Trest_def : Inport  Port=2  OutDataTypeStr=uint16  PortDimensions=1
  SimpleModeling_c4_sqCkIiGJ54r4u5oiueanYzC_node_aut : Stateflow chart  TreatAsAtomicUnit=on
  Active : Outport
  state : Outport  Port=2
  path_timer : Outport  Port=3
  wires:
  SimpleModeling_c4_sqCkIiGJ54r4u5oiueanYzC_node_aut/3(path_timer) -> path_timer/1
  SimpleModeling_c4_sqCkIiGJ54r4u5oiueanYzC_node_aut/2(state) -> state/1
  SimpleModeling_c4_sqCkIiGJ54r4u5oiueanYzC_node_aut/1(Active) -> Active/1
  Trest_def/1 -> SimpleModeling_c4_sqCkIiGJ54r4u5oiueanYzC_node_aut/2(Trest_def)
  inActive/1 -> SimpleModeling_c4_sqCkIiGJ54r4u5oiueanYzC_node_aut/1(inActive)

== system gm_case2mod_new/PA1_1to2/path_aut ==
  inActive1 : Inport  OutDataTypeStr=boolean  PortDimensions=1  SampleTime=1
  inActive2 : Inport  Port=2  OutDataTypeStr=boolean  PortDimensions=1  SampleTime=1
  forw_param : Inport  Port=3  OutDataTypeStr=uint16  PortDimensions=1
  pathTimerEn : Inport  Port=4  OutDataTypeStr=uint16  PortDimensions=1  SampleTime=1
  pathTimerEx : Inport  Port=5  OutDataTypeStr=uint16  PortDimensions=1  SampleTime=1
  SimpleModeling_c5_sKnV4uZPaUgSl9dvj35Gf4B_path_aut : Stateflow chart  TreatAsAtomicUnit=on
  outActive1 : Outport
  outActive2 : Outport  Port=2
  state : Outport  Port=3
  wires:
  inActive1/1 -> SimpleModeling_c5_sKnV4uZPaUgSl9dvj35Gf4B_path_aut/1(inActive1)
  inActive2/1 -> SimpleModeling_c5_sKnV4uZPaUgSl9dvj35Gf4B_path_aut/2(inActive2)
  forw_param/1 -> SimpleModeling_c5_sKnV4uZPaUgSl9dvj35Gf4B_path_aut/3(forw_param)
  pathTimerEn/1 -> SimpleModeling_c5_sKnV4uZPaUgSl9dvj35Gf4B_path_aut/4(pathTimerEn)
  pathTimerEx/1 -> SimpleModeling_c5_sKnV4uZPaUgSl9dvj35Gf4B_path_aut/5(pathTimerEx)
  SimpleModeling_c5_sKnV4uZPaUgSl9dvj35Gf4B_path_aut/1(outActive1) -> outActive1/1
  SimpleModeling_c5_sKnV4uZPaUgSl9dvj35Gf4B_path_aut/2(outActive2) -> outActive2/1
  SimpleModeling_c5_sKnV4uZPaUgSl9dvj35Gf4B_path_aut/3(state) -> state/1

== system gm_case2mod_new/PA2_2to3/path_aut ==
  inActive1 : Inport  OutDataTypeStr=boolean  PortDimensions=1  SampleTime=1
  inActive2 : Inport  Port=2  OutDataTypeStr=boolean  PortDimensions=1  SampleTime=1
  forw_param : Inport  Port=3  OutDataTypeStr=uint16  PortDimensions=1  SampleTime=1
  pathTimerEn : Inport  Port=4  OutDataTypeStr=uint16  PortDimensions=1  SampleTime=1
  pathTimerEx : Inport  Port=5  OutDataTypeStr=uint16  PortDimensions=1  SampleTime=1
  SimpleModeling_c5_spnshronzZ8815nA14cRtO_path_aut : Stateflow chart  TreatAsAtomicUnit=on
  outActive1 : Outport
  outActive2 : Outport  Port=2
  state : Outport  Port=3
  wires:
  inActive1/1 -> SimpleModeling_c5_spnshronzZ8815nA14cRtO_path_aut/1(inActive1)
  inActive2/1 -> SimpleModeling_c5_spnshronzZ8815nA14cRtO_path_aut/2(inActive2)
  forw_param/1 -> SimpleModeling_c5_spnshronzZ8815nA14cRtO_path_aut/3(forw_param)
  pathTimerEn/1 -> SimpleModeling_c5_spnshronzZ8815nA14cRtO_path_aut/4(pathTimerEn)
  pathTimerEx/1 -> SimpleModeling_c5_spnshronzZ8815nA14cRtO_path_aut/5(pathTimerEx)
  SimpleModeling_c5_spnshronzZ8815nA14cRtO_path_aut/1(outActive1) -> outActive1/1
  SimpleModeling_c5_spnshronzZ8815nA14cRtO_path_aut/2(outActive2) -> outActive2/1
  SimpleModeling_c5_spnshronzZ8815nA14cRtO_path_aut/3(state) -> state/1

== system gm_case2mod_new/PA3_1to4/path_aut ==
  inActive1 : Inport  OutDataTypeStr=boolean  PortDimensions=1  SampleTime=1
  inActive2 : Inport  Port=2  OutDataTypeStr=boolean  PortDimensions=1  SampleTime=1
  forw_param : Inport  Port=3  OutDataTypeStr=uint16  PortDimensions=1
  pathTimerEn : Inport  Port=4  OutDataTypeStr=uint16  PortDimensions=1  SampleTime=1
  pathTimerEx : Inport  Port=5  OutDataTypeStr=uint16  PortDimensions=1  SampleTime=1
  SimpleModeling_c5_sLRpbKPPZaNK4eVsSRGul3D_path_aut : Stateflow chart  TreatAsAtomicUnit=on
  outActive1 : Outport
  outActive2 : Outport  Port=2
  state : Outport  Port=3
  wires:
  inActive1/1 -> SimpleModeling_c5_sLRpbKPPZaNK4eVsSRGul3D_path_aut/1(inActive1)
  inActive2/1 -> SimpleModeling_c5_sLRpbKPPZaNK4eVsSRGul3D_path_aut/2(inActive2)
  forw_param/1 -> SimpleModeling_c5_sLRpbKPPZaNK4eVsSRGul3D_path_aut/3(forw_param)
  pathTimerEn/1 -> SimpleModeling_c5_sLRpbKPPZaNK4eVsSRGul3D_path_aut/4(pathTimerEn)
  pathTimerEx/1 -> SimpleModeling_c5_sLRpbKPPZaNK4eVsSRGul3D_path_aut/5(pathTimerEx)
  SimpleModeling_c5_sLRpbKPPZaNK4eVsSRGul3D_path_aut/1(outActive1) -> outActive1/1
  SimpleModeling_c5_sLRpbKPPZaNK4eVsSRGul3D_path_aut/2(outActive2) -> outActive2/1
  SimpleModeling_c5_sLRpbKPPZaNK4eVsSRGul3D_path_aut/3(state) -> state/1

== system gm_case2mod_new/PA4_1to6/path_aut ==
  inActive1 : Inport  OutDataTypeStr=boolean  PortDimensions=1  SampleTime=1
  inActive2 : Inport  Port=2  OutDataTypeStr=boolean  PortDimensions=1  SampleTime=1
  forw_param : Inport  Port=3  OutDataTypeStr=uint16  PortDimensions=1
  pathTimerEn : Inport  Port=4  OutDataTypeStr=uint16  PortDimensions=1  SampleTime=1
  pathTimerEx : Inport  Port=5  OutDataTypeStr=uint16  PortDimensions=1  SampleTime=1
  SimpleModeling_c5_sKsWQe5Kdh9JFwwvtW0IE3D_path_aut : Stateflow chart  TreatAsAtomicUnit=on
  outActive1 : Outport
  outActive2 : Outport  Port=2
  state : Outport  Port=3
  wires:
  inActive1/1 -> SimpleModeling_c5_sKsWQe5Kdh9JFwwvtW0IE3D_path_aut/1(inActive1)
  inActive2/1 -> SimpleModeling_c5_sKsWQe5Kdh9JFwwvtW0IE3D_path_aut/2(inActive2)
  forw_param/1 -> SimpleModeling_c5_sKsWQe5Kdh9JFwwvtW0IE3D_path_aut/3(forw_param)
  pathTimerEn/1 -> SimpleModeling_c5_sKsWQe5Kdh9JFwwvtW0IE3D_path_aut/4(pathTimerEn)
  pathTimerEx/1 -> SimpleModeling_c5_sKsWQe5Kdh9JFwwvtW0IE3D_path_aut/5(pathTimerEx)
  SimpleModeling_c5_sKsWQe5Kdh9JFwwvtW0IE3D_path_aut/1(outActive1) -> outActive1/1
  SimpleModeling_c5_sKsWQe5Kdh9JFwwvtW0IE3D_path_aut/2(outActive2) -> outActive2/1
  SimpleModeling_c5_sKsWQe5Kdh9JFwwvtW0IE3D_path_aut/3(state) -> state/1

== system gm_case2mod_new/PA5_4to5/path_aut ==
  inActive1 : Inport  OutDataTypeStr=boolean  PortDimensions=1  SampleTime=1
  inActive2 : Inport  Port=2  OutDataTypeStr=boolean  PortDimensions=1  SampleTime=1
  forw_param : Inport  Port=3  OutDataTypeStr=uint16  PortDimensions=1
  pathTimerEn : Inport  Port=4  OutDataTypeStr=uint16  PortDimensions=1  SampleTime=1
  pathTimerEx : Inport  Port=5  OutDataTypeStr=uint16  PortDimensions=1  SampleTime=1
  SimpleModeling_c5_s5eks8Qa0EkC2gggO4am9GG_path_aut : Stateflow chart  TreatAsAtomicUnit=on
  outActive1 : Outport
  outActive2 : Outport  Port=2
  state : Outport  Port=3
  wires:
  inActive1/1 -> SimpleModeling_c5_s5eks8Qa0EkC2gggO4am9GG_path_aut/1(inActive1)
  inActive2/1 -> SimpleModeling_c5_s5eks8Qa0EkC2gggO4am9GG_path_aut/2(inActive2)
  forw_param/1 -> SimpleModeling_c5_s5eks8Qa0EkC2gggO4am9GG_path_aut/3(forw_param)
  pathTimerEn/1 -> SimpleModeling_c5_s5eks8Qa0EkC2gggO4am9GG_path_aut/4(pathTimerEn)
  pathTimerEx/1 -> SimpleModeling_c5_s5eks8Qa0EkC2gggO4am9GG_path_aut/5(pathTimerEx)
  SimpleModeling_c5_s5eks8Qa0EkC2gggO4am9GG_path_aut/1(outActive1) -> outActive1/1
  SimpleModeling_c5_s5eks8Qa0EkC2gggO4am9GG_path_aut/2(outActive2) -> outActive2/1
  SimpleModeling_c5_s5eks8Qa0EkC2gggO4am9GG_path_aut/3(state) -> state/1

== system gm_case2mod_new/PA6_6to7/path_aut ==
  inActive1 : Inport  OutDataTypeStr=boolean  PortDimensions=1  SampleTime=1
  inActive2 : Inport  Port=2  OutDataTypeStr=boolean  PortDimensions=1  SampleTime=1
  forw_param : Inport  Port=3  OutDataTypeStr=uint16  PortDimensions=1
  pathTimerEn : Inport  Port=4  OutDataTypeStr=uint16  PortDimensions=1  SampleTime=1
  pathTimerEx : Inport  Port=5  OutDataTypeStr=uint16  PortDimensions=1  SampleTime=1
  SimpleModeling_c5_s5XQ586iC6QEN0xQSpsem4E_path_aut : Stateflow chart  TreatAsAtomicUnit=on
  outActive1 : Outport
  outActive2 : Outport  Port=2
  state : Outport  Port=3
  wires:
  inActive1/1 -> SimpleModeling_c5_s5XQ586iC6QEN0xQSpsem4E_path_aut/1(inActive1)
  inActive2/1 -> SimpleModeling_c5_s5XQ586iC6QEN0xQSpsem4E_path_aut/2(inActive2)
  forw_param/1 -> SimpleModeling_c5_s5XQ586iC6QEN0xQSpsem4E_path_aut/3(forw_param)
  pathTimerEn/1 -> SimpleModeling_c5_s5XQ586iC6QEN0xQSpsem4E_path_aut/4(pathTimerEn)
  pathTimerEx/1 -> SimpleModeling_c5_s5XQ586iC6QEN0xQSpsem4E_path_aut/5(pathTimerEx)
  SimpleModeling_c5_s5XQ586iC6QEN0xQSpsem4E_path_aut/1(outActive1) -> outActive1/1
  SimpleModeling_c5_s5XQ586iC6QEN0xQSpsem4E_path_aut/2(outActive2) -> outActive2/1
  SimpleModeling_c5_s5XQ586iC6QEN0xQSpsem4E_path_aut/3(state) -> state/1

== system gm_case2mod_new/PA7_5to7/path_aut ==
  inActive1 : Inport  OutDataTypeStr=boolean  PortDimensions=1  SampleTime=1
  inActive2 : Inport  Port=2  OutDataTypeStr=boolean  PortDimensions=1  SampleTime=1
  forw_param : Inport  Port=3  OutDataTypeStr=uint16  PortDimensions=1
  pathTimerEn : Inport  Port=4  OutDataTypeStr=uint16  PortDimensions=1  SampleTime=1
  pathTimerEx : Inport  Port=5  OutDataTypeStr=uint16  PortDimensions=1  SampleTime=1
  SimpleModeling_c5_sqcjkKS4oBcaRaS68Vk5pPE_path_aut : Stateflow chart  TreatAsAtomicUnit=on
  outActive1 : Outport
  outActive2 : Outport  Port=2
  state : Outport  Port=3
  wires:
  inActive1/1 -> SimpleModeling_c5_sqcjkKS4oBcaRaS68Vk5pPE_path_aut/1(inActive1)
  inActive2/1 -> SimpleModeling_c5_sqcjkKS4oBcaRaS68Vk5pPE_path_aut/2(inActive2)
  forw_param/1 -> SimpleModeling_c5_sqcjkKS4oBcaRaS68Vk5pPE_path_aut/3(forw_param)
  pathTimerEn/1 -> SimpleModeling_c5_sqcjkKS4oBcaRaS68Vk5pPE_path_aut/4(pathTimerEn)
  pathTimerEx/1 -> SimpleModeling_c5_sqcjkKS4oBcaRaS68Vk5pPE_path_aut/5(pathTimerEx)
  SimpleModeling_c5_sqcjkKS4oBcaRaS68Vk5pPE_path_aut/1(outActive1) -> outActive1/1
  SimpleModeling_c5_sqcjkKS4oBcaRaS68Vk5pPE_path_aut/2(outActive2) -> outActive2/1
  SimpleModeling_c5_sqcjkKS4oBcaRaS68Vk5pPE_path_aut/3(state) -> state/1

== stateflow chart gm_case2mod_new/NA2_AV/node_aut/SimpleModeling_c4_sQ0mRpZY21gn33BKqBQ1TvG_node_aut ==
  settings: executeAtInitialization=1
  state NodeAutomaton
    state RRP
      du: TRRP_cur = TRRP_cur-1;
      du: state=3;
    state Rest
      du: Trest_cur = Trest_cur-1;
      du: state=1;
    state ERP
      ex: Active = 0;
      du: TERP_cur = TERP_cur-1;
      du: path_timer = 0;
      du: Active = 0;
      du: state=2;
    (default) -> Rest : {Active=0;
        | Trest_cur = Trest_s;TERP_def=TERP_defs;
        | TERP_cur = TERP_s;
        | TRRP_cur = TRRP_s;
        | path_timer = 0;}
    RRP -> Rest [order 2] : [(~inActive) & (TRRP_cur==0)]
        | {TRRP_cur = TRRP_def;
        | path_timer = 0;}
    Rest -> ERP [order 2] : [inActive]
        | {Trest_cur = Trest_def;
        | TERP_def = Terp_max;
        | TERP_cur = Terp_max;
        | path_timer = 1;}
    Rest -> ERP [order 1] : [(~inActive) & (Trest_cur==0)]
        | {Trest_cur = Trest_def;
        | Active = 1;
        | path_timer = 0;}
    RRP -> ERP [order 1] : [inActive]
        | {TERP_def = Terp_min;
        | path_timer = 3;
        | TERP_cur = TERP_def;
        | TRRP_cur = TRRP_def;}
    ERP -> RRP [order 2] : [(~inActive) & (TERP_cur==0)]
        | {TERP_cur = TERP_def;
        | path_timer = 0;}
    ERP -> ERP [order 1] : [inActive]
        | {TERP_cur = Terp_min;
        | TERP_def = Terp_min;
        | path_timer = 3;}
  data: TERP_cur local uint16; TRRP_cur local uint16; Trest_cur local uint16; TRRP_def constant uint16 =TRRP_def_m; Active output boolean; inActive input boolean; Trest_def input uint16 =Trest_def_m; TERP_defs constant uint16 =TERP_defs_m; TERP_s constant uint16 =TERP_s_m; TRRP_s constant uint16 =TRRP_s_m; Trest_s constant uint16 =Trest_s_m; Terp_min constant uint16 =Terp_min_m; Terp_max constant uint16 =Terp_max_m; TERP_def local uint16; state output uint8; path_timer output uint16; ratio local uint16

== stateflow chart gm_case2mod_new/NA3_RV/node_aut/SimpleModeling_c4_sppf4LupdbMSnBPpv0jGkfF_node_aut ==
  settings: executeAtInitialization=1
  state NodeAutomaton
    state RRP
      du: TRRP_cur = TRRP_cur-1;
      du: state=3;
    state Rest
      du: Trest_cur = Trest_cur-1;
      du: state=1;
    state ERP
      ex: Active = 0;
      du: TERP_cur = TERP_cur-1;
      du: path_timer = 0;
      du: Active = 0;
      du: state=2;
    (default) -> Rest : {Active=0;
        | Trest_cur = Trest_s;TERP_def=TERP_defs;
        | TERP_cur = TERP_s;
        | TRRP_cur = TRRP_s;
        | path_timer = 0;}
    RRP -> Rest [order 2] : [(~inActive) & (TRRP_cur==0)]
        | {TRRP_cur = TRRP_def;
        | path_timer = 0;}
    Rest -> ERP [order 2] : [inActive]
        | {Trest_cur = Trest_def;
        | TERP_def = Terp_max;
        | TERP_cur = Terp_max;
        | path_timer = 1;}
    Rest -> ERP [order 1] : [(~inActive) & (Trest_cur==0)]
        | {Trest_cur = Trest_def;
        | Active = 1;
        | path_timer = 0;}
    RRP -> ERP [order 1] : [inActive]
        | {TERP_def = Terp_min;
        | path_timer = 3;
        | TERP_cur = TERP_def;
        | TRRP_cur = TRRP_def;}
    ERP -> RRP [order 2] : [(~inActive) & (TERP_cur==0)]
        | {TERP_cur = TERP_def;
        | path_timer = 0;}
    ERP -> ERP [order 1] : [inActive]
        | {TERP_cur = Terp_min;
        | TERP_def = Terp_min;
        | path_timer = 3;}
  data: TERP_cur local uint16; TRRP_cur local uint16; Trest_cur local uint16; TRRP_def constant uint16 =TRRP_def_m; Active output boolean; inActive input boolean; Trest_def input uint16 =Trest_def_m; TERP_defs constant uint16 =TERP_defs_m; TERP_s constant uint16 =TERP_s_m; TRRP_s constant uint16 =TRRP_s_m; Trest_s constant uint16 =Trest_s_m; Terp_min constant uint16 =Terp_min_m; Terp_max constant uint16 =Terp_max_m; TERP_def local uint16; state output uint8; path_timer output uint16; ratio local uint16

== stateflow chart gm_case2mod_new/NA4_F1/node_aut/SimpleModeling_c4_sppf4LupdbMSnBPpv0jGkfF_node_aut ==
  settings: executeAtInitialization=1
  state NodeAutomaton
    state RRP
      du: TRRP_cur = TRRP_cur-1;
      du: state=3;
    state Rest
      du: Trest_cur = Trest_cur-1;
      du: state=1;
    state ERP
      ex: Active = 0;
      du: TERP_cur = TERP_cur-1;
      du: path_timer = 0;
      du: Active = 0;
      du: state=2;
    (default) -> Rest : {Active=0;
        | Trest_cur = Trest_s;TERP_def=TERP_defs;
        | TERP_cur = TERP_s;
        | TRRP_cur = TRRP_s;
        | path_timer = 0;}
    RRP -> Rest [order 2] : [(~inActive) & (TRRP_cur==0)]
        | {TRRP_cur = TRRP_def;
        | path_timer = 0;}
    Rest -> ERP [order 2] : [inActive]
        | {Trest_cur = Trest_def;
        | TERP_def = Terp_max;
        | TERP_cur = Terp_max;
        | path_timer = 1;}
    Rest -> ERP [order 1] : [(~inActive) & (Trest_cur==0)]
        | {Trest_cur = Trest_def;
        | Active = 1;
        | path_timer = 0;}
    RRP -> ERP [order 1] : [inActive]
        | {TERP_def = Terp_min;
        | path_timer = 3;
        | TERP_cur = TERP_def;
        | TRRP_cur = TRRP_def;}
    ERP -> RRP [order 2] : [(~inActive) & (TERP_cur==0)]
        | {TERP_cur = TERP_def;
        | path_timer = 0;}
    ERP -> ERP [order 1] : [inActive]
        | {TERP_cur = Terp_min;
        | TERP_def = Terp_min;
        | path_timer = 3;}
  data: TERP_cur local uint16; TRRP_cur local uint16; Trest_cur local uint16; TRRP_def constant uint16 =TRRP_def_m; Active output boolean; inActive input boolean; Trest_def input uint16 =Trest_def_m; TERP_defs constant uint16 =TERP_defs_m; TERP_s constant uint16 =TERP_s_m; TRRP_s constant uint16 =TRRP_s_m; Trest_s constant uint16 =Trest_s_m; Terp_min constant uint16 =Terp_min_m; Terp_max constant uint16 =Terp_max_m; TERP_def local uint16; state output uint8; path_timer output uint16; ratio local uint16

== stateflow chart gm_case2mod_new/NA1_SA/node_aut/SimpleModeling_c4_srNoRdC9XVw08QQmbgBst2F_node_aut ==
  settings: executeAtInitialization=1
  state NodeAutomaton
    state RRP
      du: TRRP_cur = TRRP_cur-1;
      du: state=3;
    state Rest
      du: Trest_cur = Trest_cur-1;
      du: state=1;
    state ERP
      ex: Active = 0;
      du: TERP_cur = TERP_cur-1;
      du: path_timer = 0;
      du: Active = 0;
      du: state=2;
    (default) -> Rest : {Active=0;
        | Trest_cur = Trest_s;TERP_def=TERP_defs;
        | TERP_cur = TERP_s;
        | TRRP_cur = TRRP_s;
        | path_timer = 0;}
    RRP -> Rest [order 2] : [(~inActive) & (TRRP_cur==0)]
        | {TRRP_cur = TRRP_def;
        | path_timer = 0;}
    Rest -> ERP [order 2] : [inActive]
        | {Trest_cur = Trest_def;
        | TERP_def = Terp_max;
        | TERP_cur = Terp_max;
        | path_timer = 1;}
    Rest -> ERP [order 1] : [(~inActive) & (Trest_cur==0)]
        | {Trest_cur = Trest_def;
        | Active = 1;
        | path_timer = 0;}
    RRP -> ERP [order 1] : [inActive]
        | {TERP_def = Terp_min;
        | path_timer = 3;
        | TERP_cur = TERP_def;
        | TRRP_cur = TRRP_def;}
    ERP -> RRP [order 2] : [(~inActive) & (TERP_cur==0)]
        | {TERP_cur = TERP_def;
        | path_timer = 0;}
    ERP -> ERP [order 1] : [inActive]
        | {TERP_cur = Terp_min;
        | TERP_def = Terp_min;
        | path_timer = 3;}
  data: TERP_cur local uint16; TRRP_cur local uint16; Trest_cur local uint16; TRRP_def constant uint16 =TRRP_def_m; Active output boolean; inActive input boolean; Trest_def input uint16 =Trest_def_m; TERP_defs constant uint16 =TERP_defs_m; TERP_s constant uint16 =TERP_s_m; TRRP_s constant uint16 =TRRP_s_m; Trest_s constant uint16 =Trest_s_m; Terp_min constant uint16 =Terp_min_m; Terp_max constant uint16 =Terp_max_m; TERP_def local uint16; state output uint8; path_timer output uint16; ratio local uint16

== stateflow chart gm_case2mod_new/NA5_F2/node_aut/SimpleModeling_c4_sppf4LupdbMSnBPpv0jGkfF_node_aut ==
  settings: executeAtInitialization=1
  state NodeAutomaton
    state RRP
      du: TRRP_cur = TRRP_cur-1;
      du: state=3;
    state Rest
      du: Trest_cur = Trest_cur-1;
      du: state=1;
    state ERP
      ex: Active = 0;
      du: TERP_cur = TERP_cur-1;
      du: path_timer = 0;
      du: Active = 0;
      du: state=2;
    (default) -> Rest : {Active=0;
        | Trest_cur = Trest_s;TERP_def=TERP_defs;
        | TERP_cur = TERP_s;
        | TRRP_cur = TRRP_s;
        | path_timer = 0;}
    RRP -> Rest [order 2] : [(~inActive) & (TRRP_cur==0)]
        | {TRRP_cur = TRRP_def;
        | path_timer = 0;}
    Rest -> ERP [order 2] : [inActive]
        | {Trest_cur = Trest_def;
        | TERP_def = Terp_max;
        | TERP_cur = Terp_max;
        | path_timer = 1;}
    Rest -> ERP [order 1] : [(~inActive) & (Trest_cur==0)]
        | {Trest_cur = Trest_def;
        | Active = 1;
        | path_timer = 0;}
    RRP -> ERP [order 1] : [inActive]
        | {TERP_def = Terp_min;
        | path_timer = 3;
        | TERP_cur = TERP_def;
        | TRRP_cur = TRRP_def;}
    ERP -> RRP [order 2] : [(~inActive) & (TERP_cur==0)]
        | {TERP_cur = TERP_def;
        | path_timer = 0;}
    ERP -> ERP [order 1] : [inActive]
        | {TERP_cur = Terp_min;
        | TERP_def = Terp_min;
        | path_timer = 3;}
  data: TERP_cur local uint16; TRRP_cur local uint16; Trest_cur local uint16; TRRP_def constant uint16 =TRRP_def_m; Active output boolean; inActive input boolean; Trest_def input uint16 =Trest_def_m; TERP_defs constant uint16 =TERP_defs_m; TERP_s constant uint16 =TERP_s_m; TRRP_s constant uint16 =TRRP_s_m; Trest_s constant uint16 =Trest_s_m; Terp_min constant uint16 =Terp_min_m; Terp_max constant uint16 =Terp_max_m; TERP_def local uint16; state output uint8; path_timer output uint16; ratio local uint16

== stateflow chart gm_case2mod_new/NA6_S1/node_aut/SimpleModeling_c4_sqCkIiGJ54r4u5oiueanYzC_node_aut ==
  settings: executeAtInitialization=1
  state NodeAutomaton
    state RRP
      du: TRRP_cur = TRRP_cur-1;
      du: state=3;
    state Rest
      du: Trest_cur = Trest_cur-1;
      du: state=1;
    state ERP
      ex: Active = 0;
      du: TERP_cur = TERP_cur-1;
      du: path_timer = 0;
      du: Active = 0;
      du: state=2;
    (default) -> Rest : {Active=0;
        | Trest_cur = Trest_s;TERP_def=TERP_defs;
        | TERP_cur = TERP_s;
        | TRRP_cur = TRRP_s;
        | path_timer = 0;}
    RRP -> Rest [order 2] : [(~inActive) & (TRRP_cur==0)]
        | {TRRP_cur = TRRP_def;
        | path_timer = 0;}
    Rest -> ERP [order 2] : [inActive]
        | {Trest_cur = Trest_def;
        | TERP_def = Terp_max;
        | TERP_cur = Terp_max;
        | path_timer = 1;}
    Rest -> ERP [order 1] : [(~inActive) & (Trest_cur==0)]
        | {Trest_cur = Trest_def;
        | Active = 1;
        | path_timer = 0;}
    RRP -> ERP [order 1] : [inActive]
        | {TERP_def = Terp_min;
        | path_timer = 3;
        | TERP_cur = TERP_def;
        | TRRP_cur = TRRP_def;}
    ERP -> RRP [order 2] : [(~inActive) & (TERP_cur==0)]
        | {TERP_cur = TERP_def;
        | path_timer = 0;}
    ERP -> ERP [order 1] : [inActive]
        | {TERP_cur = Terp_min;
        | TERP_def = Terp_min;
        | path_timer = 3;}
  data: TERP_cur local uint16; TRRP_cur local uint16; Trest_cur local uint16; TRRP_def constant uint16 =TRRP_def_m; Active output boolean; inActive input boolean; Trest_def input uint16 =Trest_def_m; TERP_defs constant uint16 =TERP_defs_m; TERP_s constant uint16 =TERP_s_m; TRRP_s constant uint16 =TRRP_s_m; Trest_s constant uint16 =Trest_s_m; Terp_min constant uint16 =Terp_min_m; Terp_max constant uint16 =Terp_max_m; TERP_def local uint16; state output uint8; path_timer output uint16; ratio local uint16
